simulink model "NewSuspensionAssembly2"  (R2025b)
settings: Solver=VariableStepAuto  StartTime=0.0  StopTime=10.0  RelTol=1e-3
model workspace: external: MATLAB File E:\matlab_files\NewSuspensionAssembly2_DataFile.m (data not in the file)
undefined symbols (not defined in the file): smiData, X, Y, Z
libraries: sm_lib x138, nesl_utility x5
(part 1 of 4)
settings Model: Creator=ABHIRAJ  LastModifiedBy=ABHIRAJ

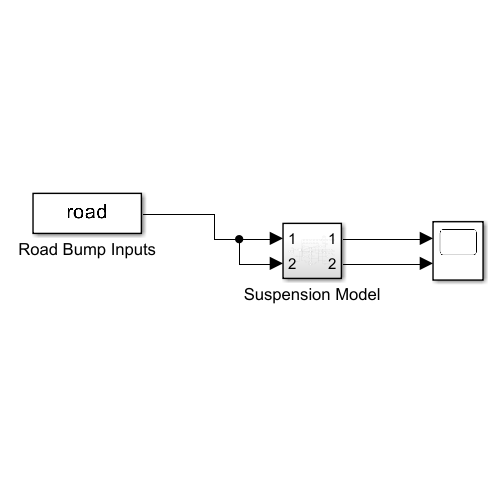
[thumbnail: Simulink's stored preview of the top-level diagram]
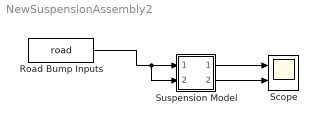
== system NewSuspensionAssembly2 ==
  Road Bump Inputs : FromWorkspace  VariableName=road
  Scope : Scope  NumInputPorts=2
      settings: ActiveDisplayYMinimum=-26227.239211791013  ActiveDisplayYMaximum=261793.07387564232
  Suspension Model : Subsystem
  wires:
  Suspension Model/1(Out2) -> Scope/1
  Road Bump Inputs/1 -> Suspension Model/2(In1), Suspension Model/1(In2)
  Suspension Model/2(Out1) -> Scope/2
